simulink model "untitled"  (R2022a)
settings: Solver=VariableStepAuto  StartTime=0.0  StopTime=10.0  RelTol=1e-3
settings Model: Creator=Андрій  LastModifiedBy=Андрій

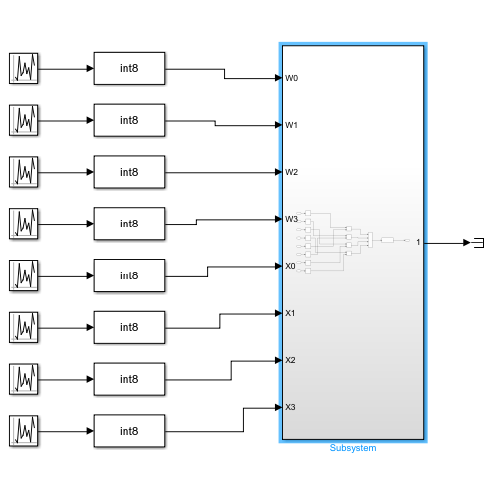
[thumbnail: Simulink's stored preview of the top-level diagram]
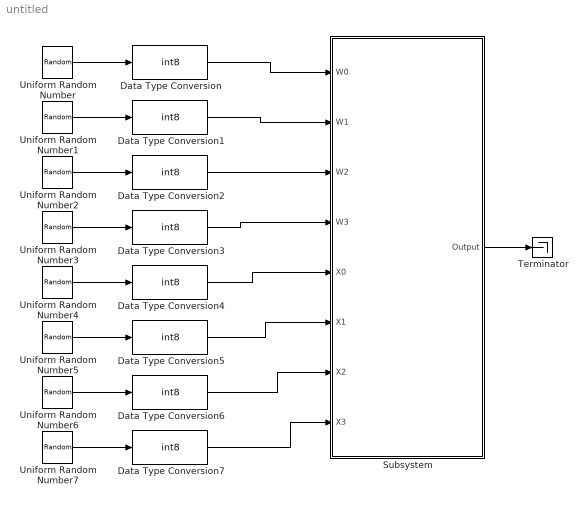
== system untitled ==
  Data Type Conversion{,1..7} (8 alike) : DataTypeConversion  OutDataTypeStr=int8  SaturateOnIntegerOverflow=off  RndMeth=Floor
  Subsystem : Subsystem
  Terminator : Terminator
  Uniform Random Number : UniformRandomNumber  Minimum=0  Maximum=2^8-1  Seed=4  SampleTime=1
  Uniform Random Number1 : UniformRandomNumber  Minimum=0  Maximum=2^8-1  Seed=5  SampleTime=1
  Uniform Random Number2 : UniformRandomNumber  Minimum=0  Maximum=2^8-1  Seed=6  SampleTime=1
  Uniform Random Number3 : UniformRandomNumber  Minimum=0  Maximum=2^8-1  Seed=7  SampleTime=1
  Uniform Random Number4 : UniformRandomNumber  Minimum=0  Maximum=2^8-1  Seed=8  SampleTime=1
  Uniform Random Number5 : UniformRandomNumber  Minimum=0  Maximum=2^8-1  Seed=9  SampleTime=1
  Uniform Random Number6 : UniformRandomNumber  Minimum=0  Maximum=2^8-1  Seed=10  SampleTime=1
  Uniform Random Number7 : UniformRandomNumber  Minimum=0  Maximum=2^8-1  Seed=11  SampleTime=1
  wires:
  Uniform Random Number/1 -> Data Type Conversion/1
  Uniform Random Number1/1 -> Data Type Conversion1/1
  Uniform Random Number2/1 -> Data Type Conversion2/1
  Uniform Random Number3/1 -> Data Type Conversion3/1
  Uniform Random Number4/1 -> Data Type Conversion4/1
  Uniform Random Number5/1 -> Data Type Conversion5/1
  Uniform Random Number6/1 -> Data Type Conversion6/1
  Uniform Random Number7/1 -> Data Type Conversion7/1
  Data Type Conversion/1 -> Subsystem/1(W0)
  Data Type Conversion1/1 -> Subsystem/2(W1)
  Data Type Conversion2/1 -> Subsystem/3(W2)
  Data Type Conversion3/1 -> Subsystem/4(W3)
  Data Type Conversion4/1 -> Subsystem/5(X0)
  Data Type Conversion5/1 -> Subsystem/6(X1)
  Data Type Conversion6/1 -> Subsystem/7(X2)
  Data Type Conversion7/1 -> Subsystem/8(X3)
  Subsystem/1(Output) -> Terminator/1

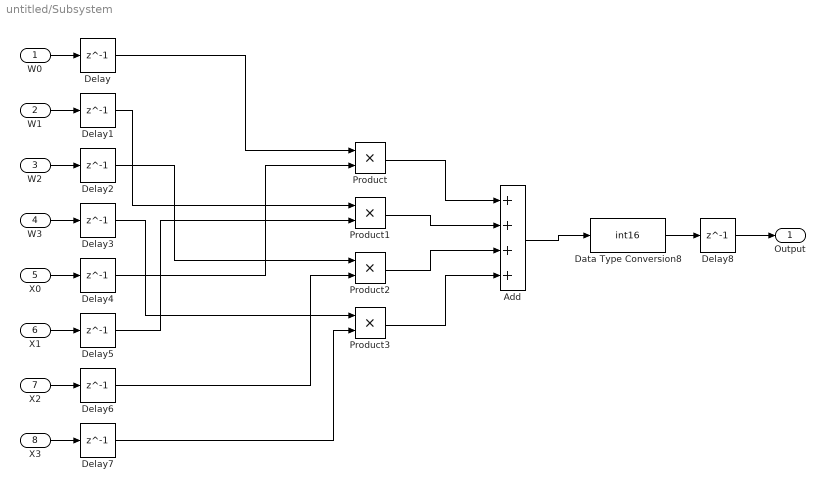
== system untitled/Subsystem ==
  W0 : Inport
  W1 : Inport  Port=2
  W2 : Inport  Port=3
  W3 : Inport  Port=4
  X0 : Inport  Port=5
  X1 : Inport  Port=6
  X2 : Inport  Port=7
  X3 : Inport  Port=8
  Add : Sum  Inputs=++++
  Data Type Conversion8 : DataTypeConversion  OutDataTypeStr=int16  SaturateOnIntegerOverflow=off  RndMeth=Floor
  Delay{,1..8} (9 alike) : Delay  DelayLength=1  InitialCondition=0
  Product{,1..3} (4 alike) : Product
  Output : Outport
  wires:
  Data Type Conversion8/1 -> Delay8/1
  Product2/1 -> Add/3
  Product/1 -> Add/1
  Add/1 -> Data Type Conversion8/1
  Product3/1 -> Add/4
  Product1/1 -> Add/2
  W0/1 -> Delay/1
  Delay/1 -> Product/1
  W1/1 -> Delay1/1
  Delay1/1 -> Product1/1
  W2/1 -> Delay2/1
  Delay2/1 -> Product2/1
  W3/1 -> Delay3/1
  Delay3/1 -> Product3/1
  X0/1 -> Delay4/1
  Delay4/1 -> Product/2
  X1/1 -> Delay5/1
  Delay5/1 -> Product1/2
  X2/1 -> Delay6/1
  Delay6/1 -> Product2/2
  X3/1 -> Delay7/1
  Delay7/1 -> Product3/2
  Delay8/1 -> Output/1
